simulink model "test_firs"  (Simulink 6.2)
settings: Solver=ode45  StartTime=0.0  StopTime=500  RelTol=1e-3
undefined symbols (not defined in the file or in its folder): now, pfb_coefs
libraries: xbsIndex_r3 x151, pfb_library x1, simulink x1
(part 2 of 3)

== system test_firs/fir/fir_tap_2 ==
  data_in : Inport  Port=1  LatchInput=off
  sum_in : Inport  Port=2  LatchInput=off
  sync_in : Inport  Port=3  LatchInput=off
  fir_coef : Subsystem  mask(FIR Filter Coefficient Generator){coef=[0.999864698373715;0.998782787093866;0.996621638554108;0.993386591798817;0.989085632941254;0.983729368318744;0.977330988864374;0.969906225835535;0.961473298073597;0.952052851002189;0.941667887603872;0.93034369164628;0.918107743458883;0.904989628590384;0.891020939704144;0.876235172094917;0.860667613234385;0.844355226775522;0.827336531466419;0.809651475442971;0.791341306386551;0.772448438047459;0.75301631364748;0.733089266685254;0.712712379676312;0.691931341365526;0.670792302953398;0.649341733878935;0.627626277701018;0.605692608616936;0.58358728915143;0.561356629541902;0.539046549335732;0.516702441703681;0.494369040959443;0.47209029375942;0.449909234438953;0.427867864921515;0.406007039615979;0.384366355693955;0.362984049114638;0.341896896738581;0.321140124844505;0.300747324334799;0.280750372885839;0.261179364268877;0.242062545036048;0.22342625873426;0.205294897777456;0.187690863075115;0.170634531482069;0.154144231101832;0.138236224442934;0.122924699395207;0.108221767960864;0.0941374726436389;0.0806798003683017;0.0678547037727424;0.0556661296856254;0.0441160545744412;0.033204526721812;0.0229297148621999;0.0132879629868503;0.00427385100197821], n_bits_c=9, bin_pt_c=8, use_bram=on}
      mask prompts: coef "Tap Coefficient(s)"; n_bits_c "Number of Coefficient Bits"; bin_pt_c "Coefficient Binary Point"; use_bram "Use BRAM for Coefficients"
      mask help: A Finite Impluse Response filter coefficient generator. This FIR filter coefficient generator outputs real coefficients. It can output one coefficient or cycle through a vector of coefficients for WOLA (Weighted OverLap Add) FIR filters.
      settings: AttributesFormatString=64 coefs in bram
      mask Help:
      | <pre>
      | Description::
      | 
      | A Finite Impluse Response filter coefficient generator.
      | This FIR filter coefficient generator outputs real coefficients.
      | It can output one coefficient or cycle through a vector of coefficients for WOLA
      | (Weighted OverLap Add) FIR filters.
      | 
      | Mask Parameters::
      | 
      | Tap Coefficiant(s) (coef): The coefficient(s) to output.  For a "regular" FIR filter, this will be a
      | single number.  For a WOLA (Weighted OverLap Add) filter, this will be a vector of numbers.
      | These should be specified as doubles.   They will be rounded and saturated according to the
      | specified number of bits (n_bits_c) and binary point (bin_pt_c).
      | 
      | Number of Coefficient Bits (n_bits_c): The number of bits used for the fixed point binary
      | representation of the coefficient(s).
      | 
      | Coefficient Binary Point (bin_pt_c): The binary point of the fixed point binary representation
      | of the coefficient(s).
      | 
      | Use BRAM for Coefficients (use_bram): Check this checkbox to store the coefficients in BRAM.
      | If unchecked, the coefficients will be stored in distributed memory (i.e. slices).
      | This is only relevant is length(coef) is greater than 1; otherwise, a constant block is used.
      | </pre>
  fir_core : Subsystem  mask(FIR Filter Core){delay=64, n_bits_d=8, bin_pt_d=7, n_bits_s=17, bin_pt_s=15, use_bram=on, mult_latency=3, add_latency=1, add_bypass=off}
      mask prompts: delay "Tap Delay"; n_bits_d "Number of Data Bits"; bin_pt_d "Data Binary Point"; n_bits_s "Number of Sum Bits"; bin_pt_s "Sum Binary Point"; use_bram "Use BRAM for Delay"; mult_latency "Multiplier Latency"; add_latency "Adder Latency"; add_bypass "Bypass Adder"
      mask help: A Finite Impluse Response Filter core with complex inputs and real coefficients. This FIR filter core does not have provisions for folding the input sequence to improve multiplier efficiency, so it is suboptimal for "regular" (i.e. non-WOLA) FIR filters. It is intended primarily for WOLA (Weighted OverLap Add) FIR filters.
      settings: AttributesFormatString=delay 64 in bram
      mask Help:
      | <pre>
      | Description::
      | 
      | A Finite Impluse Response Filter core with complex inputs and real coefficients.
      | 
      | This Finite Impluse Response Filter core is designed to be paired with a FIR Coefficient Generator
      | to form a FIR filter tap.  This FIR filter core does not have provisions for folding the input
      | sequence to improve multiplier efficiency, so it is suboptimal for "regular" (i.e. non-WOLA)
      | FIR filters.  It is intended primarily for WOLA (Weighted OverLap Add) FIR filters.
      | 
      | Mask Parameters::
      | 
      | Tap Delay (delay):  The inter-tap delay (the N in "z^-N").  For a regular FIR filter, this will be 1.
      | 
      | Number of Data Bits (n_bits_d): The number of bits for real/imaginary components of the data.
      | 
      | Data Binary Point (bin_pt_d): The binary point for real/imaginary components of the data.
      | 
      | Number of Sum Bits (n_bits_s): Specifies the width of the sum (overflow wraps).
      | 
      | Sum Binary Point (bin_pt_s): Specifies the binary point of the sum (quantization truncates).
      | 
      | Use BRAM for Delay (use_bram): Check this checkbox to implement the delay using BRAM.
      | If unchecked, the delay will be implemented using SLR16 elements (i.e. slices).
      | 
      | Multiplier Latency (mult_latency): Latency to use for the underlying multiplier.
      | 
      | Adder Latency (add_latency): Latency to use for the underlying adder.
      | 
      | Adder Bypass (add_bypass): Check this checkbox to bypass the adder.
      | Typically used for the first tap of a multi-tap FIR filter.
      | </pre>
  data_out : Outport
  sum_out : Outport  Port=2
  sync_out : Outport  Port=3
  wires:
  fir_core/3(sync_out) -> sync_out/1
  fir_core/2(sum_out) -> sum_out/1
  fir_core/1(data_out) -> data_out/1
  sync_in/1 -> fir_coef/3(sync_in)
  sum_in/1 -> fir_coef/2(sum_in)
  data_in/1 -> fir_coef/1(data_in)
  fir_coef/4(sync_out) -> fir_core/4(sync_in)
  fir_coef/3(coef) -> fir_core/3(coef)
  fir_coef/2(sum_out) -> fir_core/2(sum_in)
  fir_coef/1(data_out) -> fir_core/1(data_in)

== system test_firs/fir/fir_tap_3 ==
  data_in : Inport  Port=1  LatchInput=off
  sum_in : Inport  Port=2  LatchInput=off
  sync_in : Inport  Port=3  LatchInput=off
  fir_coef : Subsystem  mask(FIR Filter Coefficient Generator){coef=[0.00427385100197821;0.0132879629868503;0.0229297148621999;0.033204526721812;0.0441160545744412;0.0556661296856254;0.0678547037727424;0.0806798003683017;0.0941374726436389;0.108221767960864;0.122924699395207;0.138236224442934;0.154144231101832;0.170634531482069;0.187690863075115;0.205294897777456;0.22342625873426;0.242062545036048;0.261179364268877;0.280750372885839;0.300747324334799;0.321140124844505;0.341896896738581;0.362984049114638;0.384366355693955;0.406007039615979;0.427867864921515;0.449909234438953;0.47209029375942;0.494369040959443;0.516702441703681;0.539046549335732;0.561356629541902;0.58358728915143;0.605692608616936;0.627626277701018;0.649341733878935;0.670792302953398;0.691931341365526;0.712712379676312;0.733089266685254;0.75301631364748;0.772448438047459;0.791341306386551;0.809651475442971;0.827336531466419;0.844355226775522;0.860667613234385;0.876235172094917;0.891020939704144;0.904989628590384;0.918107743458883;0.93034369164628;0.941667887603872;0.952052851002189;0.961473298073597;0.969906225835535;0.977330988864374;0.983729368318744;0.989085632941254;0.993386591798817;0.996621638554108;0.998782787093866;0.999864698373715], n_bits_c=9, bin_pt_c=8, use_bram=on}
      mask prompts: coef "Tap Coefficient(s)"; n_bits_c "Number of Coefficient Bits"; bin_pt_c "Coefficient Binary Point"; use_bram "Use BRAM for Coefficients"
      mask help: A Finite Impluse Response filter coefficient generator. This FIR filter coefficient generator outputs real coefficients. It can output one coefficient or cycle through a vector of coefficients for WOLA (Weighted OverLap Add) FIR filters.
      settings: AttributesFormatString=64 coefs in bram
      mask Help:
      | <pre>
      | Description::
      | 
      | A Finite Impluse Response filter coefficient generator.
      | This FIR filter coefficient generator outputs real coefficients.
      | It can output one coefficient or cycle through a vector of coefficients for WOLA
      | (Weighted OverLap Add) FIR filters.
      | 
      | Mask Parameters::
      | 
      | Tap Coefficiant(s) (coef): The coefficient(s) to output.  For a "regular" FIR filter, this will be a
      | single number.  For a WOLA (Weighted OverLap Add) filter, this will be a vector of numbers.
      | These should be specified as doubles.   They will be rounded and saturated according to the
      | specified number of bits (n_bits_c) and binary point (bin_pt_c).
      | 
      | Number of Coefficient Bits (n_bits_c): The number of bits used for the fixed point binary
      | representation of the coefficient(s).
      | 
      | Coefficient Binary Point (bin_pt_c): The binary point of the fixed point binary representation
      | of the coefficient(s).
      | 
      | Use BRAM for Coefficients (use_bram): Check this checkbox to store the coefficients in BRAM.
      | If unchecked, the coefficients will be stored in distributed memory (i.e. slices).
      | This is only relevant is length(coef) is greater than 1; otherwise, a constant block is used.
      | </pre>
  fir_core : Subsystem  mask(FIR Filter Core){delay=64, n_bits_d=8, bin_pt_d=7, n_bits_s=17, bin_pt_s=15, use_bram=on, mult_latency=3, add_latency=1, add_bypass=off}
      mask prompts: delay "Tap Delay"; n_bits_d "Number of Data Bits"; bin_pt_d "Data Binary Point"; n_bits_s "Number of Sum Bits"; bin_pt_s "Sum Binary Point"; use_bram "Use BRAM for Delay"; mult_latency "Multiplier Latency"; add_latency "Adder Latency"; add_bypass "Bypass Adder"
      mask help: A Finite Impluse Response Filter core with complex inputs and real coefficients. This FIR filter core does not have provisions for folding the input sequence to improve multiplier efficiency, so it is suboptimal for "regular" (i.e. non-WOLA) FIR filters. It is intended primarily for WOLA (Weighted OverLap Add) FIR filters.
      settings: AttributesFormatString=delay 64 in bram
      mask Help:
      | <pre>
      | Description::
      | 
      | A Finite Impluse Response Filter core with complex inputs and real coefficients.
      | 
      | This Finite Impluse Response Filter core is designed to be paired with a FIR Coefficient Generator
      | to form a FIR filter tap.  This FIR filter core does not have provisions for folding the input
      | sequence to improve multiplier efficiency, so it is suboptimal for "regular" (i.e. non-WOLA)
      | FIR filters.  It is intended primarily for WOLA (Weighted OverLap Add) FIR filters.
      | 
      | Mask Parameters::
      | 
      | Tap Delay (delay):  The inter-tap delay (the N in "z^-N").  For a regular FIR filter, this will be 1.
      | 
      | Number of Data Bits (n_bits_d): The number of bits for real/imaginary components of the data.
      | 
      | Data Binary Point (bin_pt_d): The binary point for real/imaginary components of the data.
      | 
      | Number of Sum Bits (n_bits_s): Specifies the width of the sum (overflow wraps).
      | 
      | Sum Binary Point (bin_pt_s): Specifies the binary point of the sum (quantization truncates).
      | 
      | Use BRAM for Delay (use_bram): Check this checkbox to implement the delay using BRAM.
      | If unchecked, the delay will be implemented using SLR16 elements (i.e. slices).
      | 
      | Multiplier Latency (mult_latency): Latency to use for the underlying multiplier.
      | 
      | Adder Latency (add_latency): Latency to use for the underlying adder.
      | 
      | Adder Bypass (add_bypass): Check this checkbox to bypass the adder.
      | Typically used for the first tap of a multi-tap FIR filter.
      | </pre>
  data_out : Outport
  sum_out : Outport  Port=2
  sync_out : Outport  Port=3
  wires:
  fir_core/3(sync_out) -> sync_out/1
  fir_core/2(sum_out) -> sum_out/1
  fir_core/1(data_out) -> data_out/1
  sync_in/1 -> fir_coef/3(sync_in)
  sum_in/1 -> fir_coef/2(sum_in)
  data_in/1 -> fir_coef/1(data_in)
  fir_coef/4(sync_out) -> fir_core/4(sync_in)
  fir_coef/3(coef) -> fir_core/3(coef)
  fir_coef/2(sum_out) -> fir_core/2(sum_in)
  fir_coef/1(data_out) -> fir_core/1(data_in)

== system test_firs/fir/fir_tap_4 ==
  data_in : Inport  Port=1  LatchInput=off
  sum_in : Inport  Port=2  LatchInput=off
  sync_in : Inport  Port=3  LatchInput=off
  fir_coef : Subsystem  mask(FIR Filter Coefficient Generator){coef=[-0.000313693993479576;-0.000949413894136895;-0.00160072502983972;-0.00227308910223182;-0.00297201531120363;-0.00370300584524142;-0.00447149996896613;-0.00528281700660057;-0.0061420985300509;-0.0070542500687595;-0.00802388266542662;-0.00905525460705801;-0.0101522136645361;-0.0113181401759998;-0.0125558913097251;-0.0138677468409146;-0.0152553567738119;-0.0167196911358607;-0.018260992264242;-0.0198787298970449;-0.0215715593716044;-0.0233372832211883;-0.0251728164482839;-0.0270741557382724;-0.0290363528613422;-0.0310534924931389;-0.0331186746659681;-0.035224002042413;-0.0373605721821118;-0.039518474950235;-0.0416867951930131;-0.0438536207815986;-0.0460060561007039;-0.0481302410329562;-0.050211375463868;-0.0522337493058552;-0.0541807780129703;-0.0560350435310833;-0.057778340601254;-0.0593917283071436;-0.0608555867306188;-0.0621496785533557;-0.063253215416367;-0.0641449288240917;-0.064803145355121;-0.0652058659179099;-0.0653308487670656;-0.0651556959741166;-0.0646579430261756;-0.0638151512067052;-0.0626050023947942;-0.0610053959030371;-0.0589945469593747;-0.0565510864251856;-0.0536541613305752;-0.0502835357982813;-0.0464196919199395;-0.0420439301426944;-0.0371384687203353;-0.03168654178132;-0.0256724955662416;-0.0190818823895147;-0.0119015518843096;-0.00411973909604202], n_bits_c=9, bin_pt_c=8, use_bram=on}
      mask prompts: coef "Tap Coefficient(s)"; n_bits_c "Number of Coefficient Bits"; bin_pt_c "Coefficient Binary Point"; use_bram "Use BRAM for Coefficients"
      mask help: A Finite Impluse Response filter coefficient generator. This FIR filter coefficient generator outputs real coefficients. It can output one coefficient or cycle through a vector of coefficients for WOLA (Weighted OverLap Add) FIR filters.
      settings: AttributesFormatString=64 coefs in bram
      mask Help:
      | <pre>
      | Description::
      | 
      | A Finite Impluse Response filter coefficient generator.
      | This FIR filter coefficient generator outputs real coefficients.
      | It can output one coefficient or cycle through a vector of coefficients for WOLA
      | (Weighted OverLap Add) FIR filters.
      | 
      | Mask Parameters::
      | 
      | Tap Coefficiant(s) (coef): The coefficient(s) to output.  For a "regular" FIR filter, this will be a
      | single number.  For a WOLA (Weighted OverLap Add) filter, this will be a vector of numbers.
      | These should be specified as doubles.   They will be rounded and saturated according to the
      | specified number of bits (n_bits_c) and binary point (bin_pt_c).
      | 
      | Number of Coefficient Bits (n_bits_c): The number of bits used for the fixed point binary
      | representation of the coefficient(s).
      | 
      | Coefficient Binary Point (bin_pt_c): The binary point of the fixed point binary representation
      | of the coefficient(s).
      | 
      | Use BRAM for Coefficients (use_bram): Check this checkbox to store the coefficients in BRAM.
      | If unchecked, the coefficients will be stored in distributed memory (i.e. slices).
      | This is only relevant is length(coef) is greater than 1; otherwise, a constant block is used.
      | </pre>
  fir_core : Subsystem  mask(FIR Filter Core){delay=0, n_bits_d=8, bin_pt_d=7, n_bits_s=17, bin_pt_s=15, use_bram=off, mult_latency=3, add_latency=1, add_bypass=off}
      mask prompts: delay "Tap Delay"; n_bits_d "Number of Data Bits"; bin_pt_d "Data Binary Point"; n_bits_s "Number of Sum Bits"; bin_pt_s "Sum Binary Point"; use_bram "Use BRAM for Delay"; mult_latency "Multiplier Latency"; add_latency "Adder Latency"; add_bypass "Bypass Adder"
      mask help: A Finite Impluse Response Filter core with complex inputs and real coefficients. This FIR filter core does not have provisions for folding the input sequence to improve multiplier efficiency, so it is suboptimal for "regular" (i.e. non-WOLA) FIR filters. It is intended primarily for WOLA (Weighted OverLap Add) FIR filters.
      settings: AttributesFormatString=delay 0 in slr
      mask Help:
      | <pre>
      | Description::
      | 
      | A Finite Impluse Response Filter core with complex inputs and real coefficients.
      | 
      | This Finite Impluse Response Filter core is designed to be paired with a FIR Coefficient Generator
      | to form a FIR filter tap.  This FIR filter core does not have provisions for folding the input
      | sequence to improve multiplier efficiency, so it is suboptimal for "regular" (i.e. non-WOLA)
      | FIR filters.  It is intended primarily for WOLA (Weighted OverLap Add) FIR filters.
      | 
      | Mask Parameters::
      | 
      | Tap Delay (delay):  The inter-tap delay (the N in "z^-N").  For a regular FIR filter, this will be 1.
      | 
      | Number of Data Bits (n_bits_d): The number of bits for real/imaginary components of the data.
      | 
      | Data Binary Point (bin_pt_d): The binary point for real/imaginary components of the data.
      | 
      | Number of Sum Bits (n_bits_s): Specifies the width of the sum (overflow wraps).
      | 
      | Sum Binary Point (bin_pt_s): Specifies the binary point of the sum (quantization truncates).
      | 
      | Use BRAM for Delay (use_bram): Check this checkbox to implement the delay using BRAM.
      | If unchecked, the delay will be implemented using SLR16 elements (i.e. slices).
      | 
      | Multiplier Latency (mult_latency): Latency to use for the underlying multiplier.
      | 
      | Adder Latency (add_latency): Latency to use for the underlying adder.
      | 
      | Adder Bypass (add_bypass): Check this checkbox to bypass the adder.
      | Typically used for the first tap of a multi-tap FIR filter.
      | </pre>
  data_out : Outport
  sum_out : Outport  Port=2
  sync_out : Outport  Port=3
  wires:
  fir_core/3(sync_out) -> sync_out/1
  fir_core/2(sum_out) -> sum_out/1
  fir_core/1(data_out) -> data_out/1
  sync_in/1 -> fir_coef/3(sync_in)
  sum_in/1 -> fir_coef/2(sum_in)
  data_in/1 -> fir_coef/1(data_in)
  fir_coef/4(sync_out) -> fir_core/4(sync_in)
  fir_coef/3(coef) -> fir_core/3(coef)
  fir_coef/2(sum_out) -> fir_core/2(sum_in)
  fir_coef/1(data_out) -> fir_core/1(data_in)

== system test_firs/fir/fir_quantize/c_to_ri ==
  c : Inport  Port=1  LatchInput=off
  force_im : xbsIndex_r3/Reinterpret  force_arith_type=on  arith_type="Signed  (2's comp)"  force_bin_pt=on  bin_pt=15  force_valid=on
  force_re : xbsIndex_r3/Reinterpret  force_arith_type=on  arith_type="Signed  (2's comp)"  force_bin_pt=on  bin_pt=15  force_valid=on
  slice_im : xbsIndex_r3/Slice  mode=Lower Bit Location + Width  nbits=17  bit1=0  base1=MSB of Input  bit0=0  base0=LSB of Input  boolean_output=off  explicit_period=off  period=1  dbl_ovrd=off
  slice_re : xbsIndex_r3/Slice  mode=Upper Bit Location + Width  nbits=17  bit1=0  base1=MSB of Input  bit0=0  base0=LSB of Input  boolean_output=off  explicit_period=off  period=1  dbl_ovrd=off
  re : Outport
  im : Outport  Port=2
  wires:
  slice_re/1 -> force_re/1
  slice_im/1 -> force_im/1
  force_re/1 -> re/1
  force_im/1 -> im/1
  c/1 -> slice_re/1, slice_im/1

== system test_firs/fir/fir_quantize/ri_to_c ==
  re : Inport  Port=1  LatchInput=off
  im : Inport  Port=2  LatchInput=off
  concat : xbsIndex_r3/Concat  num_inputs=2  explicit_period=off  period=1  dbl_ovrd=off
  force_im : xbsIndex_r3/Reinterpret  force_arith_type=on  arith_type=Unsigned  force_bin_pt=on  bin_pt=0  force_valid=on
  force_re : xbsIndex_r3/Reinterpret  force_arith_type=on  arith_type=Unsigned  force_bin_pt=on  bin_pt=0  force_valid=on
  c : Outport
  wires:
  im/1 -> force_im/1
  concat/1 -> c/1
  re/1 -> force_re/1
  force_im/1 -> concat/2
  force_re/1 -> concat/1

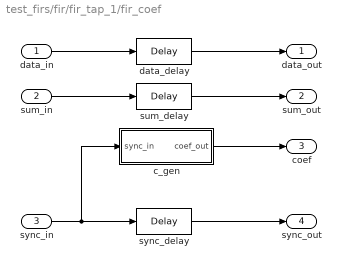
== system test_firs/fir/fir_tap_1/fir_coef ==
  data_in : Inport  Port=1  LatchInput=off
  sum_in : Inport  Port=2  LatchInput=off
  sync_in : Inport  Port=3  LatchInput=off
  c_gen : Subsystem  mask(Coefficient Generator){coefs=[-0.00411973909604202;-0.0119015518843096;-0.0190818823895147;-0.0256724955662416;-0.03168654178132;-0.0371384687203353;-0.0420439301426944;-0.0464196919199395;-0.0502835357982813;-0.0536541613305752;-0.0565510864251856;-0.0589945469593747;-0.0610053959030371;-0.0626050023947942;-0.0638151512067052;-0.0646579430261756;-0.0651556959741166;-0.0653308487670656;-0.0652058659179099;-0.064803145355121;-0.0641449288240917;-0.063253215416367;-0.0621496785533557;-0.0608555867306188;-0.0593917283071436;-0.057778340601254;-0.0560350435310833;-0.0541807780129703;-0.0522337493058552;-0.050211375463868;-0.0481302410329562;-0.0460060561007039;-0.0438536207815986;-0.0416867951930131;-0.039518474950235;-0.0373605721821118;-0.035224002042413;-0.0331186746659681;-0.0310534924931389;-0.0290363528613422;-0.0270741557382724;-0.0251728164482839;-0.0233372832211883;-0.0215715593716044;-0.0198787298970449;-0.018260992264242;-0.0167196911358607;-0.0152553567738119;-0.0138677468409146;-0.0125558913097251;-0.0113181401759998;-0.0101522136645361;-0.00905525460705801;-0.00802388266542662;-0.0070542500687595;-0.0061420985300509;-0.00528281700660057;-0.00447149996896613;-0.00370300584524142;-0.00297201531120363;-0.00227308910223182;-0.00160072502983972;-0.000949413894136895;-0.000313693993479576], n_bits=9, bin_pt=8, log2_cpc=0, use_bram=on}
      mask prompts: coefs "Coefficients"; n_bits "Number of Bits"; bin_pt "Binary Point"; log2_cpc "Log2 Cycles per Coefficient"; use_bram "Use BRAM"
      mask help: A coefficient generator.
      settings: AttributesFormatString=|
      | 64 coefs in bram
      | 9_8 out/1
      mask Help:
      | <pre>
      | Description::
      | 
      | A coefficient generator.
      | 
      | Mask Parameters::
      | 
      | Coefficiants (coefs): The coefficients to output.  These should be specified as doubles.
      | They will be rounded/saturated according to the specified number of bits (n_bits)
      | and binary point (bin_pt).
      | 
      | Number of Coefficient Bits (n_bits): The number of bits used for the fixed point binary
      | representation of the coefficients.
      | 
      | Coefficient Binary Point (bin_pt): The binary point of the fixed point binary representation
      | of the coefficients.
      | 
      | Log2 Cycles per Coefficient (log2_cpc): The log2 value of the number of cycles per coefficient.
      | Must be a non-negative integer (i.e. cycles per coefficient must be a power of 2).
      | 
      | Use BRAM (use_bram): Check this checkbox to store coefficients in BRAM.
      | If unchecked, the coefficients will be sored in distributed memory (i.e. slices).
      | </pre>
  data_delay : xbsIndex_r3/Delay  latency=1  reg_retiming=off  explicit_period=off  period=1  en=off  accept_only_valid=off  init_zero=on  dbl_ovrd=off  show_param=on
      settings: xl_area=[0, 0, 0, 0, 0, 0, 0]
  sum_delay : xbsIndex_r3/Delay  latency=1  reg_retiming=off  explicit_period=off  period=1  en=off  accept_only_valid=off  init_zero=on  dbl_ovrd=off  show_param=on
      settings: xl_area=[0, 0, 0, 0, 0, 0, 0]
  sync_delay : xbsIndex_r3/Delay  latency=1  reg_retiming=off  explicit_period=off  period=1  en=off  accept_only_valid=off  init_zero=on  dbl_ovrd=off  show_param=off
      settings: xl_area=[0, 0, 0, 0, 0, 0, 0]
  data_out : Outport
  sum_out : Outport  Port=2
  coef : Outport  Port=3
  sync_out : Outport  Port=4
  wires:
  c_gen/1(coef_out) -> coef/1
  sum_delay/1 -> sum_out/1
  sum_in/1 -> sum_delay/1
  sync_in/1 -> c_gen/1(sync_in), sync_delay/1
  sync_delay/1 -> sync_out/1
  data_delay/1 -> data_out/1
  data_in/1 -> data_delay/1

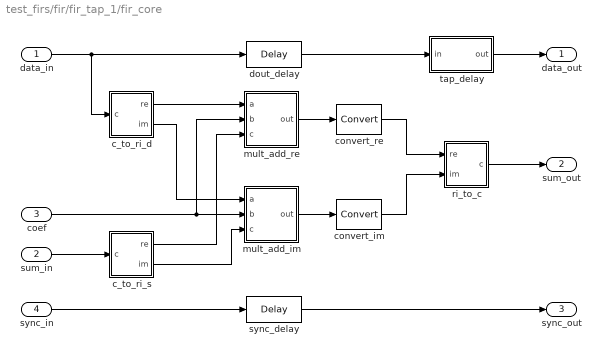
== system test_firs/fir/fir_tap_1/fir_core ==
  data_in : Inport  Port=1  LatchInput=off
  sum_in : Inport  Port=2  LatchInput=off
  coef : Inport  Port=3  LatchInput=off
  sync_in : Inport  Port=4  LatchInput=off
  c_to_ri_d : Subsystem  mask(Complex to Real-Imag){n_bits=8, bin_pt=7}
      mask prompts: n_bits "Bit Width"; bin_pt "Binary Point"
      mask help: Outputs real and imaginary components of a complex input.
      settings: AttributesFormatString=8_7 r/i
      mask Help:
      | <pre>
      | Description::
      | 
      | Outputs real and imaginary components of a complex input.
      | Useful for simplifying interconnects.
      | See also: Real-Imag to Complex (ri_to_c)
      | 
      | Mask Parameters::
      | 
      | Bit Width (n_bits): Specifies the width of the real/imaginary components.
      | Assumed equal for both components.
      | 
      | Binary Point (bin_pt): Specifies the binary point location in the real/imaginary components.
      | Assumed equal for both components.
      | </pre>
  c_to_ri_s : Subsystem  mask(Complex to Real-Imag){n_bits=17, bin_pt=15}
      mask prompts: n_bits "Bit Width"; bin_pt "Binary Point"
      mask help: Outputs real and imaginary components of a complex input.
      settings: AttributesFormatString=17_15 r/i
      mask Help:
      | <pre>
      | Description::
      | 
      | Outputs real and imaginary components of a complex input.
      | Useful for simplifying interconnects.
      | See also: Real-Imag to Complex (ri_to_c)
      | 
      | Mask Parameters::
      | 
      | Bit Width (n_bits): Specifies the width of the real/imaginary components.
      | Assumed equal for both components.
      | 
      | Binary Point (bin_pt): Specifies the binary point location in the real/imaginary components.
      | Assumed equal for both components.
      | </pre>
  convert_im : xbsIndex_r3/Convert  arith_type="Signed  (2's comp)"  n_bits=17  bin_pt=15  quantization=Truncate  overflow=Wrap  latency=0  explicit_period=off  period=1  dbl_ovrd=off  show_param=on  inserted_by_tool=off  pipeline=on
      settings: xl_area=[0, 0, 0, 0, 0, 0, 0]
  convert_re : xbsIndex_r3/Convert  arith_type="Signed  (2's comp)"  n_bits=17  bin_pt=15  quantization=Truncate  overflow=Wrap  latency=0  explicit_period=off  period=1  dbl_ovrd=off  show_param=on  inserted_by_tool=off  pipeline=on
      settings: xl_area=[0, 0, 0, 0, 0, 0, 0]
  dout_delay : xbsIndex_r3/Delay  latency=3  reg_retiming=off  explicit_period=off  period=1  en=off  accept_only_valid=off  init_zero=on  dbl_ovrd=off  show_param=off
      settings: xl_area=[0, 0, 0, 0, 0, 0, 0]
  mult_add_im : Subsystem  mask(Multiply Add Block){mult_latency=3, add_latency=1, add_bypass=on}
      mask prompts: mult_latency "Multiplier Latency"; add_latency "Adder Latency"; add_bypass "Bypass Adder"
      mask help: A full precision multiply-add block. Produces a*b+c at its ab_c output. The add operation can be optionally bypassed.
      settings: AttributesFormatString=|
      | out = a*b
      | latency = 3
      mask Help:
      | <pre>
      | Description::
      | 
      | This full precision multiply-add block produces a*b+c at its ab_c output.
      | The add operation can be optionally bypassed.
      | 
      | Latency is one multiplier latency plus one adder latency (if not bypassing adder).
      | 
      | Mask Parameters::
      | 
      | Multiplier Latency (mult_latency): Latency to use for the underlying real multipliers.
      | 
      | Adder Latency (add_latency): Latency to use for the underlying real adders.
      | 
      | Bypass Adder (add_bypass): Check this checkbox to bypass the adder.
      | </pre>
  mult_add_re : Subsystem  mask(Multiply Add Block){mult_latency=3, add_latency=1, add_bypass=on}
      mask prompts: mult_latency "Multiplier Latency"; add_latency "Adder Latency"; add_bypass "Bypass Adder"
      mask help: A full precision multiply-add block. Produces a*b+c at its ab_c output. The add operation can be optionally bypassed.
      settings: AttributesFormatString=|
      | out = a*b
      | latency = 3
      mask Help:
      | <pre>
      | Description::
      | 
      | This full precision multiply-add block produces a*b+c at its ab_c output.
      | The add operation can be optionally bypassed.
      | 
      | Latency is one multiplier latency plus one adder latency (if not bypassing adder).
      | 
      | Mask Parameters::
      | 
      | Multiplier Latency (mult_latency): Latency to use for the underlying real multipliers.
      | 
      | Adder Latency (add_latency): Latency to use for the underlying real adders.
      | 
      | Bypass Adder (add_bypass): Check this checkbox to bypass the adder.
      | </pre>
  ri_to_c : Subsystem  mask(Real-Imag to Complex){}
      mask help: Concatenates real and imaginary inputs into a complex output.
      mask init:
      | ri_to_c_init(gcb);
      mask Help:
      | <pre>
      | Description::
      | 
      | Concatenates a real and imaginary input into a complex output.
      | Useful for simplifying interconnects.
      | See also: Complex to Real-Imag (c_to_ri)
      | 
      | Mask Parameters::
      | 
      | (N/A)
      | </pre>
  sync_delay : xbsIndex_r3/Delay  latency=3  reg_retiming=off  explicit_period=off  period=1  en=off  accept_only_valid=off  init_zero=on  dbl_ovrd=off  show_param=off
      settings: xl_area=[0, 0, 0, 0, 0, 0, 0]
  tap_delay : Subsystem  mask(BRAM Delay){delay_depth=64, buffer_latency=}
      mask prompts: delay_depth "Delay Depth"; buffer_latency "Buffer Latency"
      mask help: A delay block that uses BRAM for its storage.
      settings: AttributesFormatString=bram depth = 64
      mask Help:
      | <pre>
      | Description::
      | 
      | A delay block that uses BRAM for its storage.
      | 
      | Mask Parameters::
      | 
      | Delay Depth (delay_depth): The length of the delay.
      | 
      | Buffer Latency (buffer_latency): The latency of the underlying storage.
      | 
      | Buffer Latency defaults to 1 and cannot be changed via the block's dialog box.
      | Future versions may enable the setting of that parameter from the dialog.
      | </pre>
  data_out : Outport
  sum_out : Outport  Port=2
  sync_out : Outport  Port=3
  wires:
  convert_im/1 -> ri_to_c/2(im)
  convert_re/1 -> ri_to_c/1(re)
  tap_delay/1(out) -> data_out/1
  mult_add_im/1(out) -> convert_im/1
  mult_add_re/1(out) -> convert_re/1
  c_to_ri_s/2(im) -> mult_add_im/3(c)
  c_to_ri_s/1(re) -> mult_add_re/3(c)
  sum_in/1 -> c_to_ri_s/1(c)
  coef/1 -> mult_add_re/2(b), mult_add_im/2(b)
  c_to_ri_d/2(im) -> mult_add_im/1(a)
  c_to_ri_d/1(re) -> mult_add_re/1(a)
  data_in/1 -> c_to_ri_d/1(c), dout_delay/1
  dout_delay/1 -> tap_delay/1(in)
  ri_to_c/1(c) -> sum_out/1
  sync_delay/1 -> sync_out/1
  sync_in/1 -> sync_delay/1

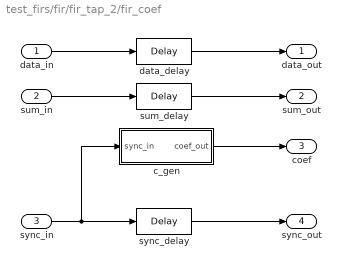
== system test_firs/fir/fir_tap_2/fir_coef ==
  data_in : Inport  Port=1  LatchInput=off
  sum_in : Inport  Port=2  LatchInput=off
  sync_in : Inport  Port=3  LatchInput=off
  c_gen : Subsystem  mask(Coefficient Generator){coefs=[0.999864698373715;0.998782787093866;0.996621638554108;0.993386591798817;0.989085632941254;0.983729368318744;0.977330988864374;0.969906225835535;0.961473298073597;0.952052851002189;0.941667887603872;0.93034369164628;0.918107743458883;0.904989628590384;0.891020939704144;0.876235172094917;0.860667613234385;0.844355226775522;0.827336531466419;0.809651475442971;0.791341306386551;0.772448438047459;0.75301631364748;0.733089266685254;0.712712379676312;0.691931341365526;0.670792302953398;0.649341733878935;0.627626277701018;0.605692608616936;0.58358728915143;0.561356629541902;0.539046549335732;0.516702441703681;0.494369040959443;0.47209029375942;0.449909234438953;0.427867864921515;0.406007039615979;0.384366355693955;0.362984049114638;0.341896896738581;0.321140124844505;0.300747324334799;0.280750372885839;0.261179364268877;0.242062545036048;0.22342625873426;0.205294897777456;0.187690863075115;0.170634531482069;0.154144231101832;0.138236224442934;0.122924699395207;0.108221767960864;0.0941374726436389;0.0806798003683017;0.0678547037727424;0.0556661296856254;0.0441160545744412;0.033204526721812;0.0229297148621999;0.0132879629868503;0.00427385100197821], n_bits=9, bin_pt=8, log2_cpc=0, use_bram=on}
      mask prompts: coefs "Coefficients"; n_bits "Number of Bits"; bin_pt "Binary Point"; log2_cpc "Log2 Cycles per Coefficient"; use_bram "Use BRAM"
      mask help: A coefficient generator.
      settings: AttributesFormatString=|
      | 64 coefs in bram
      | 9_8 out/1
      mask Help:
      | <pre>
      | Description::
      | 
      | A coefficient generator.
      | 
      | Mask Parameters::
      | 
      | Coefficiants (coefs): The coefficients to output.  These should be specified as doubles.
      | They will be rounded/saturated according to the specified number of bits (n_bits)
      | and binary point (bin_pt).
      | 
      | Number of Coefficient Bits (n_bits): The number of bits used for the fixed point binary
      | representation of the coefficients.
      | 
      | Coefficient Binary Point (bin_pt): The binary point of the fixed point binary representation
      | of the coefficients.
      | 
      | Log2 Cycles per Coefficient (log2_cpc): The log2 value of the number of cycles per coefficient.
      | Must be a non-negative integer (i.e. cycles per coefficient must be a power of 2).
      | 
      | Use BRAM (use_bram): Check this checkbox to store coefficients in BRAM.
      | If unchecked, the coefficients will be sored in distributed memory (i.e. slices).
      | </pre>
  data_delay : xbsIndex_r3/Delay  latency=1  reg_retiming=off  explicit_period=off  period=1  en=off  accept_only_valid=off  init_zero=on  dbl_ovrd=off  show_param=on
      settings: xl_area=[0, 0, 0, 0, 0, 0, 0]
  sum_delay : xbsIndex_r3/Delay  latency=1  reg_retiming=off  explicit_period=off  period=1  en=off  accept_only_valid=off  init_zero=on  dbl_ovrd=off  show_param=on
      settings: xl_area=[0, 0, 0, 0, 0, 0, 0]
  sync_delay : xbsIndex_r3/Delay  latency=1  reg_retiming=off  explicit_period=off  period=1  en=off  accept_only_valid=off  init_zero=on  dbl_ovrd=off  show_param=off
      settings: xl_area=[0, 0, 0, 0, 0, 0, 0]
  data_out : Outport
  sum_out : Outport  Port=2
  coef : Outport  Port=3
  sync_out : Outport  Port=4
  wires:
  c_gen/1(coef_out) -> coef/1
  sum_delay/1 -> sum_out/1
  sum_in/1 -> sum_delay/1
  sync_in/1 -> c_gen/1(sync_in), sync_delay/1
  sync_delay/1 -> sync_out/1
  data_delay/1 -> data_out/1
  data_in/1 -> data_delay/1

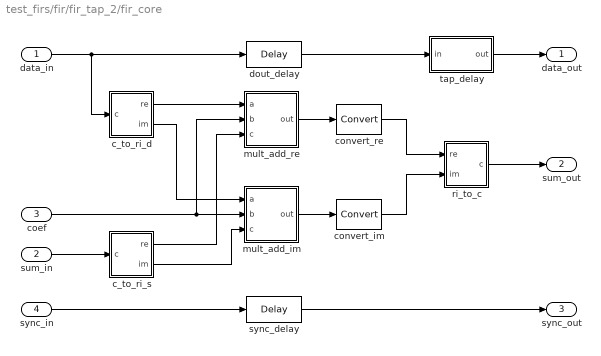
== system test_firs/fir/fir_tap_2/fir_core ==
  data_in : Inport  Port=1  LatchInput=off
  sum_in : Inport  Port=2  LatchInput=off
  coef : Inport  Port=3  LatchInput=off
  sync_in : Inport  Port=4  LatchInput=off
  c_to_ri_d : Subsystem  mask(Complex to Real-Imag){n_bits=8, bin_pt=7}
      mask prompts: n_bits "Bit Width"; bin_pt "Binary Point"
      mask help: Outputs real and imaginary components of a complex input.
      settings: AttributesFormatString=8_7 r/i
      mask Help:
      | <pre>
      | Description::
      | 
      | Outputs real and imaginary components of a complex input.
      | Useful for simplifying interconnects.
      | See also: Real-Imag to Complex (ri_to_c)
      | 
      | Mask Parameters::
      | 
      | Bit Width (n_bits): Specifies the width of the real/imaginary components.
      | Assumed equal for both components.
      | 
      | Binary Point (bin_pt): Specifies the binary point location in the real/imaginary components.
      | Assumed equal for both components.
      | </pre>
  c_to_ri_s : Subsystem  mask(Complex to Real-Imag){n_bits=17, bin_pt=15}
      mask prompts: n_bits "Bit Width"; bin_pt "Binary Point"
      mask help: Outputs real and imaginary components of a complex input.
      settings: AttributesFormatString=17_15 r/i
      mask Help:
      | <pre>
      | Description::
      | 
      | Outputs real and imaginary components of a complex input.
      | Useful for simplifying interconnects.
      | See also: Real-Imag to Complex (ri_to_c)
      | 
      | Mask Parameters::
      | 
      | Bit Width (n_bits): Specifies the width of the real/imaginary components.
      | Assumed equal for both components.
      | 
      | Binary Point (bin_pt): Specifies the binary point location in the real/imaginary components.
      | Assumed equal for both components.
      | </pre>
  convert_im : xbsIndex_r3/Convert  arith_type="Signed  (2's comp)"  n_bits=17  bin_pt=15  quantization=Truncate  overflow=Wrap  latency=0  explicit_period=off  period=1  dbl_ovrd=off  show_param=on  inserted_by_tool=off  pipeline=on
      settings: xl_area=[0, 0, 0, 0, 0, 0, 0]
  convert_re : xbsIndex_r3/Convert  arith_type="Signed  (2's comp)"  n_bits=17  bin_pt=15  quantization=Truncate  overflow=Wrap  latency=0  explicit_period=off  period=1  dbl_ovrd=off  show_param=on  inserted_by_tool=off  pipeline=on
      settings: xl_area=[0, 0, 0, 0, 0, 0, 0]
  dout_delay : xbsIndex_r3/Delay  latency=4  reg_retiming=off  explicit_period=off  period=1  en=off  accept_only_valid=off  init_zero=on  dbl_ovrd=off  show_param=off
      settings: xl_area=[0, 0, 0, 0, 0, 0, 0]
  mult_add_im : Subsystem  mask(Multiply Add Block){mult_latency=3, add_latency=1, add_bypass=off}
      mask prompts: mult_latency "Multiplier Latency"; add_latency "Adder Latency"; add_bypass "Bypass Adder"
      mask help: A full precision multiply-add block. Produces a*b+c at its ab_c output. The add operation can be optionally bypassed.
      settings: AttributesFormatString=|
      | out = a*b+c
      | latency = 4
      mask Help:
      | <pre>
      | Description::
      | 
      | This full precision multiply-add block produces a*b+c at its ab_c output.
      | The add operation can be optionally bypassed.
      | 
      | Latency is one multiplier latency plus one adder latency (if not bypassing adder).
      | 
      | Mask Parameters::
      | 
      | Multiplier Latency (mult_latency): Latency to use for the underlying real multipliers.
      | 
      | Adder Latency (add_latency): Latency to use for the underlying real adders.
      | 
      | Bypass Adder (add_bypass): Check this checkbox to bypass the adder.
      | </pre>
  mult_add_re : Subsystem  mask(Multiply Add Block){mult_latency=3, add_latency=1, add_bypass=off}
      mask prompts: mult_latency "Multiplier Latency"; add_latency "Adder Latency"; add_bypass "Bypass Adder"
      mask help: A full precision multiply-add block. Produces a*b+c at its ab_c output. The add operation can be optionally bypassed.
      settings: AttributesFormatString=|
      | out = a*b+c
      | latency = 4
      mask Help:
      | <pre>
      | Description::
      | 
      | This full precision multiply-add block produces a*b+c at its ab_c output.
      | The add operation can be optionally bypassed.
      | 
      | Latency is one multiplier latency plus one adder latency (if not bypassing adder).
      | 
      | Mask Parameters::
      | 
      | Multiplier Latency (mult_latency): Latency to use for the underlying real multipliers.
      | 
      | Adder Latency (add_latency): Latency to use for the underlying real adders.
      | 
      | Bypass Adder (add_bypass): Check this checkbox to bypass the adder.
      | </pre>
  ri_to_c : Subsystem  mask(Real-Imag to Complex){}
      mask help: Concatenates real and imaginary inputs into a complex output.
      mask init:
      | ri_to_c_init(gcb);
      mask Help:
      | <pre>
      | Description::
      | 
      | Concatenates a real and imaginary input into a complex output.
      | Useful for simplifying interconnects.
      | See also: Complex to Real-Imag (c_to_ri)
      | 
      | Mask Parameters::
      | 
      | (N/A)
      | </pre>
  sync_delay : xbsIndex_r3/Delay  latency=4  reg_retiming=off  explicit_period=off  period=1  en=off  accept_only_valid=off  init_zero=on  dbl_ovrd=off  show_param=off
      settings: xl_area=[0, 0, 0, 0, 0, 0, 0]
  tap_delay : Subsystem  mask(BRAM Delay){delay_depth=64, buffer_latency=}
      mask prompts: delay_depth "Delay Depth"; buffer_latency "Buffer Latency"
      mask help: A delay block that uses BRAM for its storage.
      settings: AttributesFormatString=bram depth = 64
      mask Help:
      | <pre>
      | Description::
      | 
      | A delay block that uses BRAM for its storage.
      | 
      | Mask Parameters::
      | 
      | Delay Depth (delay_depth): The length of the delay.
      | 
      | Buffer Latency (buffer_latency): The latency of the underlying storage.
      | 
      | Buffer Latency defaults to 1 and cannot be changed via the block's dialog box.
      | Future versions may enable the setting of that parameter from the dialog.
      | </pre>
  data_out : Outport
  sum_out : Outport  Port=2
  sync_out : Outport  Port=3
  wires:
  convert_im/1 -> ri_to_c/2(im)
  convert_re/1 -> ri_to_c/1(re)
  tap_delay/1(out) -> data_out/1
  mult_add_im/1(out) -> convert_im/1
  mult_add_re/1(out) -> convert_re/1
  c_to_ri_s/2(im) -> mult_add_im/3(c)
  c_to_ri_s/1(re) -> mult_add_re/3(c)
  sum_in/1 -> c_to_ri_s/1(c)
  coef/1 -> mult_add_re/2(b), mult_add_im/2(b)
  c_to_ri_d/2(im) -> mult_add_im/1(a)
  c_to_ri_d/1(re) -> mult_add_re/1(a)
  data_in/1 -> c_to_ri_d/1(c), dout_delay/1
  dout_delay/1 -> tap_delay/1(in)
  ri_to_c/1(c) -> sum_out/1
  sync_delay/1 -> sync_out/1
  sync_in/1 -> sync_delay/1

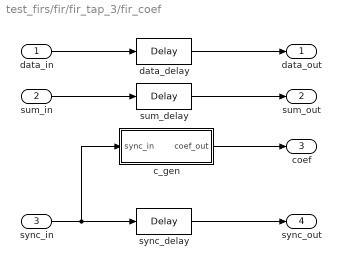
== system test_firs/fir/fir_tap_3/fir_coef ==
  data_in : Inport  Port=1  LatchInput=off
  sum_in : Inport  Port=2  LatchInput=off
  sync_in : Inport  Port=3  LatchInput=off
  c_gen : Subsystem  mask(Coefficient Generator){coefs=[0.00427385100197821;0.0132879629868503;0.0229297148621999;0.033204526721812;0.0441160545744412;0.0556661296856254;0.0678547037727424;0.0806798003683017;0.0941374726436389;0.108221767960864;0.122924699395207;0.138236224442934;0.154144231101832;0.170634531482069;0.187690863075115;0.205294897777456;0.22342625873426;0.242062545036048;0.261179364268877;0.280750372885839;0.300747324334799;0.321140124844505;0.341896896738581;0.362984049114638;0.384366355693955;0.406007039615979;0.427867864921515;0.449909234438953;0.47209029375942;0.494369040959443;0.516702441703681;0.539046549335732;0.561356629541902;0.58358728915143;0.605692608616936;0.627626277701018;0.649341733878935;0.670792302953398;0.691931341365526;0.712712379676312;0.733089266685254;0.75301631364748;0.772448438047459;0.791341306386551;0.809651475442971;0.827336531466419;0.844355226775522;0.860667613234385;0.876235172094917;0.891020939704144;0.904989628590384;0.918107743458883;0.93034369164628;0.941667887603872;0.952052851002189;0.961473298073597;0.969906225835535;0.977330988864374;0.983729368318744;0.989085632941254;0.993386591798817;0.996621638554108;0.998782787093866;0.999864698373715], n_bits=9, bin_pt=8, log2_cpc=0, use_bram=on}
      mask prompts: coefs "Coefficients"; n_bits "Number of Bits"; bin_pt "Binary Point"; log2_cpc "Log2 Cycles per Coefficient"; use_bram "Use BRAM"
      mask help: A coefficient generator.
      settings: AttributesFormatString=|
      | 64 coefs in bram
      | 9_8 out/1
      mask Help:
      | <pre>
      | Description::
      | 
      | A coefficient generator.
      | 
      | Mask Parameters::
      | 
      | Coefficiants (coefs): The coefficients to output.  These should be specified as doubles.
      | They will be rounded/saturated according to the specified number of bits (n_bits)
      | and binary point (bin_pt).
      | 
      | Number of Coefficient Bits (n_bits): The number of bits used for the fixed point binary
      | representation of the coefficients.
      | 
      | Coefficient Binary Point (bin_pt): The binary point of the fixed point binary representation
      | of the coefficients.
      | 
      | Log2 Cycles per Coefficient (log2_cpc): The log2 value of the number of cycles per coefficient.
      | Must be a non-negative integer (i.e. cycles per coefficient must be a power of 2).
      | 
      | Use BRAM (use_bram): Check this checkbox to store coefficients in BRAM.
      | If unchecked, the coefficients will be sored in distributed memory (i.e. slices).
      | </pre>
  data_delay : xbsIndex_r3/Delay  latency=1  reg_retiming=off  explicit_period=off  period=1  en=off  accept_only_valid=off  init_zero=on  dbl_ovrd=off  show_param=on
      settings: xl_area=[0, 0, 0, 0, 0, 0, 0]
  sum_delay : xbsIndex_r3/Delay  latency=1  reg_retiming=off  explicit_period=off  period=1  en=off  accept_only_valid=off  init_zero=on  dbl_ovrd=off  show_param=on
      settings: xl_area=[0, 0, 0, 0, 0, 0, 0]
  sync_delay : xbsIndex_r3/Delay  latency=1  reg_retiming=off  explicit_period=off  period=1  en=off  accept_only_valid=off  init_zero=on  dbl_ovrd=off  show_param=off
      settings: xl_area=[0, 0, 0, 0, 0, 0, 0]
  data_out : Outport
  sum_out : Outport  Port=2
  coef : Outport  Port=3
  sync_out : Outport  Port=4
  wires:
  c_gen/1(coef_out) -> coef/1
  sum_delay/1 -> sum_out/1
  sum_in/1 -> sum_delay/1
  sync_in/1 -> c_gen/1(sync_in), sync_delay/1
  sync_delay/1 -> sync_out/1
  data_delay/1 -> data_out/1
  data_in/1 -> data_delay/1
